simulink model "robot_dynamics"  (R2017a)
settings: Solver=VariableStepAuto  StartTime=0.0  StopTime=10.0  RelTol=1e-3
values from neighbouring files (symbols this model uses):
  D1 = 7*Kp*Td*eye(3)    [PDController_Test.m]
  K1 = 5*Kp*eye(3)    [PDController_Test.m]
  mass = 10    [PDController_Test.m]    (also in makeMatrixes.m = 1)
  state = A*state + B*xdd'    [PDController_Test.m]
settings Model: Creator=nathaniel  LastModifiedBy=nathaniel

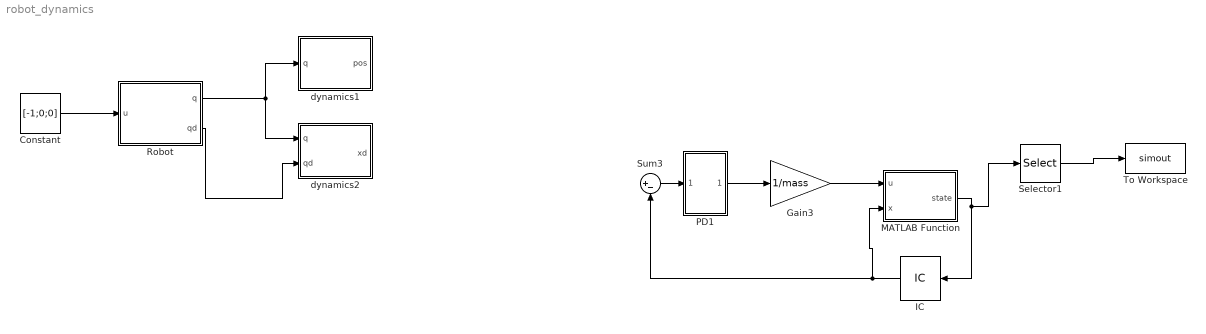
== system robot_dynamics ==
  Constant : Constant  Value=[-1;0;0]  VectorParams1D=off
  Gain3 : Gain  Gain=1/mass
  IC : InitialCondition  Value=state
  MATLAB Function : MATLAB Function  TreatAsAtomicUnit=on
  PD1 : Subsystem
  Robot : Subsystem
  Selector1 : Selector  InputPortWidth=6  IndexOptions=Index vector (dialog)  Indices=[1]  OutputSizes=1
  Sum3 : Sum  Inputs=|+-
  To Workspace : ToWorkspace  VariableName=simout  SampleTime=-1
  dynamics1 : MATLAB Function  TreatAsAtomicUnit=on
  dynamics2 : MATLAB Function  TreatAsAtomicUnit=on
  wires:
  Constant/1 -> Robot/1(u)
  Robot/1(q) -> dynamics1/1(q), dynamics2/1(q)
  Robot/2(qd) -> dynamics2/2(qd)
  Gain3/1 -> MATLAB Function/1(u)
  Sum3/1 -> PD1/1(In1)
  MATLAB Function/1(state) -> Selector1/1, IC/1
  Selector1/1 -> To Workspace/1
  PD1/1(Out1) -> Gain3/1
  IC/1 -> MATLAB Function/2(x), Sum3/2

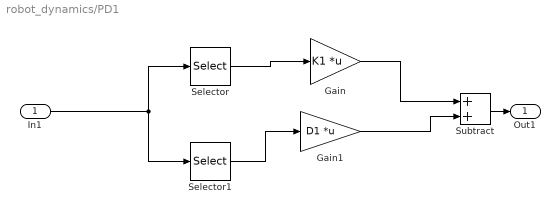
== system robot_dynamics/PD1 ==
  In1 : Inport
  Gain : Gain  Gain=K1  Multiplication=Matrix(K*u)
  Gain1 : Gain  Gain=D1  Multiplication=Matrix(K*u)
  Selector : Selector  InputPortWidth=6  IndexOptions=Index vector (dialog)  Indices=[1 2 3]  OutputSizes=1
  Selector1 : Selector  InputPortWidth=6  IndexOptions=Index vector (dialog)  Indices=[4 5 6]  OutputSizes=1
  Subtract : Sum
  Out1 : Outport
  wires:
  Gain/1 -> Subtract/1
  Selector/1 -> Gain/1
  Subtract/1 -> Out1/1
  In1/1 -> Selector/1, Selector1/1
  Gain1/1 -> Subtract/2
  Selector1/1 -> Gain1/1

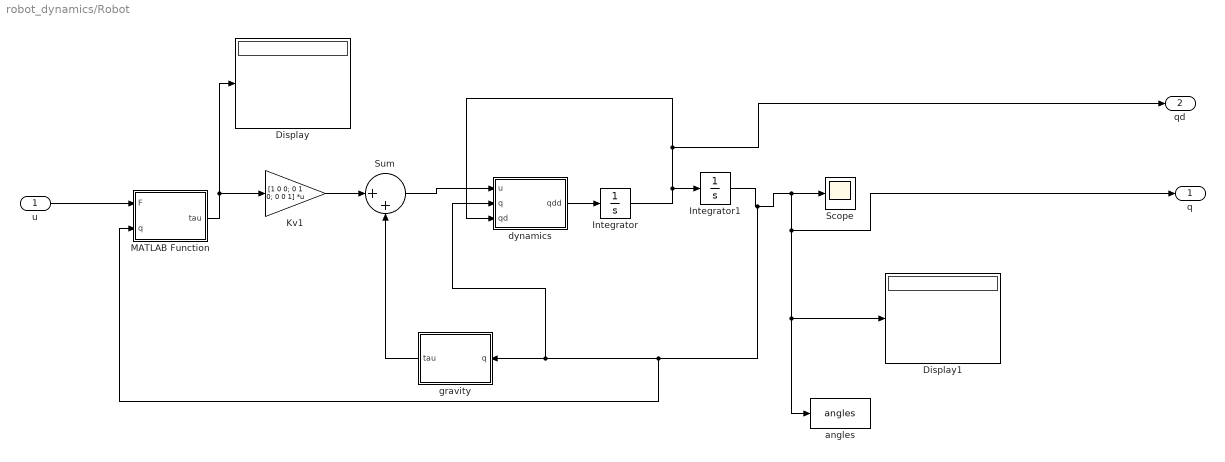
== system robot_dynamics/Robot ==
  u : Inport
  Display : Display
  Display1 : Display
  Integrator : Integrator  InitialCondition=[0;0;0]  ContinuousStateAttributes='vel'
  Integrator1 : Integrator  InitialCondition=[0;0;0]  ZeroCross=off  ContinuousStateAttributes='pos'
  Kv1 : Gain  Gain="[1 0 0; 0 1 0;  0 0 1]"  Multiplication=Matrix(K*u) (u vector)
  MATLAB Function : MATLAB Function  TreatAsAtomicUnit=on
  Scope : Scope
  Sum : Sum  Inputs=|++
  angles : ToWorkspace  VariableName=angles  SampleTime=-1
  dynamics : MATLAB Function  TreatAsAtomicUnit=on
  gravity : MATLAB Function  TreatAsAtomicUnit=on
  q : Outport
  qd : Outport  Port=2
  wires:
  dynamics/1(qdd) -> Integrator/1
  Sum/1 -> dynamics/1(u)
  MATLAB Function/1(tau) -> Display/1, Kv1/1
  Kv1/1 -> Sum/1
  gravity/1(tau) -> Sum/2
  Integrator/1 -> qd/1, dynamics/3(qd), Integrator1/1
  u/1 -> MATLAB Function/1(F)
  Integrator1/1 -> MATLAB Function/2(q), dynamics/2(q), gravity/1(q), q/1, Display1/1, angles/1, Scope/1

== matlab function robot_dynamics/Robot/MATLAB Function ==
  data: F input; tau output; q input
function tau = fcn(F,q)

    
    J = getJ(q(1),q(2),q(3))
    tau = transpose(J)*F;
end

== matlab function robot_dynamics/Robot/gravity ==
  data: q input; tau output
function tau = fcn(q)

    tau = getG(q(1),q(2),q(3));
end

== matlab function robot_dynamics/Robot/dynamics ==
  data: u input; qdd output; q input; qd input
function qdd = fcn(u,q,qd)

M = getM(q(1),q(2),q(3));
G = getG(q(1),q(2),q(3));
qdd = inv(M)*(u-G);

== matlab function robot_dynamics/dynamics1 ==
  data: pos output; q input
function pos = fcn(q)
    x = FK(q);
end

== matlab function robot_dynamics/dynamics2 ==
  data: xd output; q input; qd input
function xd = fcn(q,qd)
    xd =getJ(q)*qd;
end

== matlab function robot_dynamics/MATLAB Function ==
  data: u input; x input; state output
function state  = fcn(u,x)
dt = 0.01;
A = eye(6);

A(1:3,4:6) = dt*eye(3);
B = zeros(6,3);
D = 0*B;
C = eye(6);
B(4:6,1:3) = dt*eye(3);


state = A*x + B*u
